simulink model "EPSAC"  (R2016a)
settings: Solver=VariableStepAuto  StartTime=0.0  StopTime=5  RelTol=1e-3
libraries: powerlib x11
settings Model: Creator=jorda  LastModifiedBy=jorda

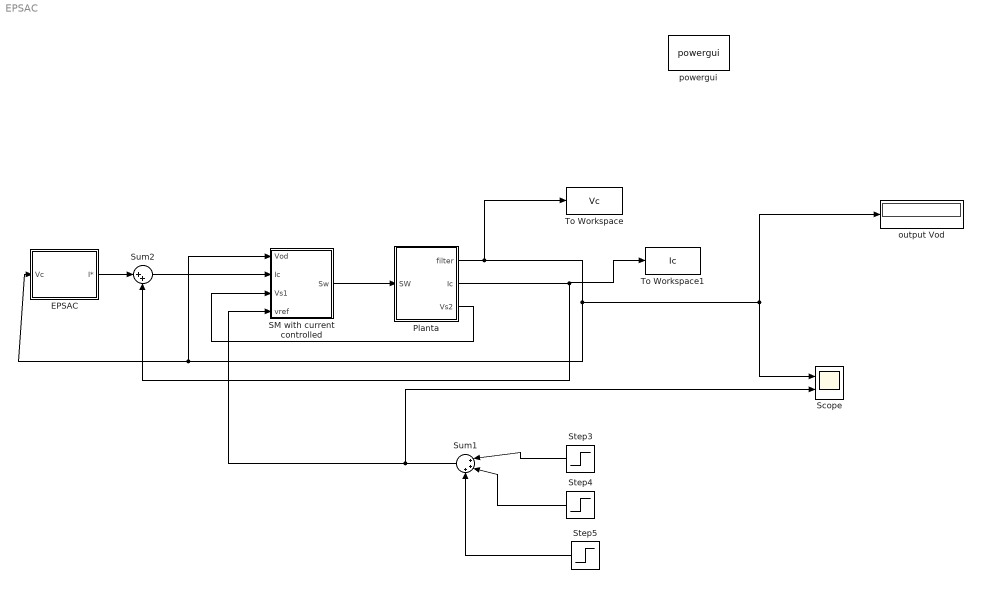
== system EPSAC ==
  EPSAC : Subsystem
  Planta : Subsystem
  SM with current controlled : Subsystem
  Scope : Scope  NumInputPorts=2
  Step3 : Step  Before=20  After=22  SampleTime=0
  Step4 : Step  Time=3  After=-2  SampleTime=0
  Step5 : Step  Time=4  Before=3  After=0  SampleTime=0
  Sum1 : Sum  Inputs=|+++
  Sum2 : Sum  Inputs=|++
  To Workspace : ToWorkspace  VariableName=Vc  SaveFormat=Timeseries  SampleTime=-1
  To Workspace1 : ToWorkspace  VariableName=Ic  SaveFormat=Timeseries  SampleTime=-1
  output Vod : Display
  powergui : powerlib/powergui  Priority=1  SimulationMode=Continuous  SolverType=Tustin/Backward Euler (TBE)  SampleTime=50e-6  frequency=60  SPID=off  DisableSnubberDevices=off  DisableRonSwitches=off  DisableVfSwitches=off  SwTol=0  DisplayEquations=off  Interpol=off  ExternalGateDelay=off  methode=off  Ts=10  FunctionMessages=off  echomessages=off  HookPort=off  EnableUseOfTLC=off  x0status=blocks  frequencyindice=0  Pbase=100e6  ErrMax=1e-4  Iterations=50  UnitsV=kV  UnitsW=MW  buscounter=0  RestoreLinks=warning  ResistiveCurrentMeasurement=off  Frange=[0:2:500]  Ylog=off  Xlog=on  ShowGrid=off  save=off  variable=ZData  structure=0  ZoomFFT=off  StartTime=0.0  cycles=1  DisplayStyle=1  fundamental=60  FreqAxis=off  MaxFrequency=1000  frequencyindicesteady=1  RmsSteady=1  display=off
  wires:
  Step3/1 -> Sum1/1
  Step4/1 -> Sum1/2
  Step5/1 -> Sum1/3
  Planta/3(Vs2) -> SM with current controlled/3("Vs1 ")
  Planta/1(filter) -> To Workspace/1, output Vod/1, Scope/1, EPSAC/1(Vc), SM with current controlled/1(Vod)
  SM with current controlled/1(Sw) -> Planta/1(SW)
  Sum2/1 -> SM with current controlled/2(Ic)
  Sum1/1 -> SM with current controlled/4(vref), Scope/2
  Planta/2(Ic) -> Sum2/2, To Workspace1/1
  EPSAC/1(I*) -> Sum2/1

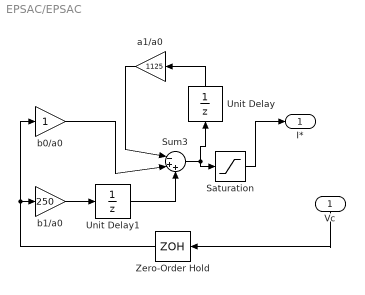
== system EPSAC/EPSAC ==
  Vc : Inport
  Saturation : Saturate  UpperLimit=0.4  LowerLimit=-0.4
  Sum3 : Sum  Inputs=|-++
  Unit Delay : UnitDelay  SampleTime=-1
  Unit Delay1 : UnitDelay  SampleTime=-1
  Zero-Order Hold : ZeroOrderHold  SampleTime=4
  a1/a0 : Gain  Gain=1125
  b0/a0 : Gain
  b1/a0 : Gain  Gain=250
  I* : Outport
  wires:
  Vc/1 -> Zero-Order Hold/1
  Saturation/1 -> I*/1
  b0/a0/1 -> Sum3/2
  Zero-Order Hold/1 -> b0/a0/1, b1/a0/1
  b1/a0/1 -> Unit Delay1/1
  Unit Delay1/1 -> Sum3/3
  a1/a0/1 -> Sum3/1
  Unit Delay/1 -> a1/a0/1
  Sum3/1 -> Saturation/1, Unit Delay/1

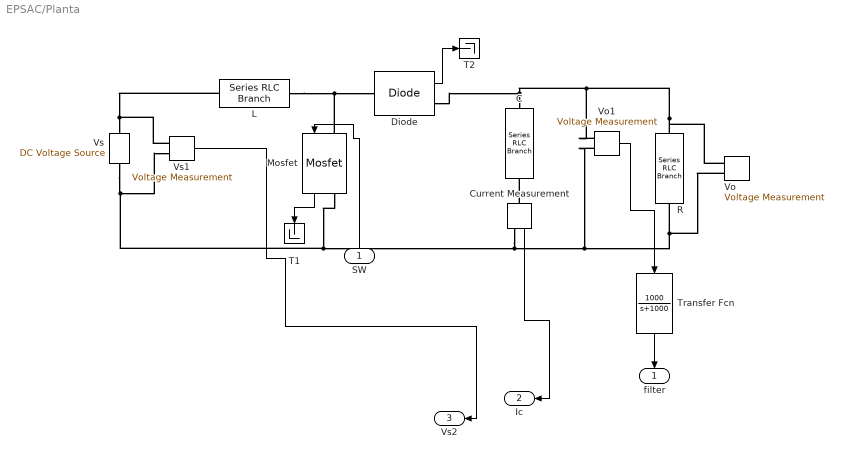
== system EPSAC/Planta ==
  SW : Inport
  C : powerlib/Elements/Series RLC Branch  LConnTagsString=__new0  RConnTagsString=__new0  BranchType=C  Resistance=1  Inductance=1e-3  SetiL0=off  InitialCurrent=0  Capacitance=2000e-6  Setx0=off  InitialVoltage=0  Measurements=None
  Current Measurement : powerlib/Measurements/Current Measurement  PhasorSimulation=off  OutputType=Complex  PSBequivalent=0
  Diode : powerlib/Power Electronics/Diode  Ron=0.001  Lon=0  Vf=0.8  IC=0  UseSnubber=off  Rs=500  Cs=250e-9  Measurements=on
  L : powerlib/Elements/Series RLC Branch  LConnTagsString=__new0  RConnTagsString=__new0  BranchType=L  Resistance=1  Inductance=2e-3  SetiL0=off  InitialCurrent=0  Capacitance=1e-6  Setx0=off  InitialVoltage=0  Measurements=None
  Mosfet : powerlib/Power Electronics/Mosfet  Ron=0.1  Lon=0  Rd=0.01  Vfd=0  IC=0  Rs=1e5  Cs=inf  Measurements=on
  R : powerlib/Elements/Series RLC Branch  LConnTagsString=__new0  RConnTagsString=__new0  BranchType=R  Resistance=4  Inductance=1e-3  SetiL0=off  InitialCurrent=0  Capacitance=1e-6  Setx0=off  InitialVoltage=0  Measurements=None
  T1 : Terminator
  T2 : Terminator
  Transfer Fcn : TransferFcn  Numerator=[1000]  Denominator=[1 1000]
  Vo : powerlib/Measurements/Voltage Measurement  PhasorSimulation=off  OutputType=Complex  PSBequivalent=0
  Vo1 : powerlib/Measurements/Voltage Measurement  PhasorSimulation=off  OutputType=Complex  PSBequivalent=0
  Vs : powerlib/Electrical Sources/DC Voltage Source  Amplitude=15  Measurements=None
  Vs1 : powerlib/Measurements/Voltage Measurement  PhasorSimulation=off  OutputType=Complex  PSBequivalent=0
  filter : Outport
  Ic : Outport  Port=2
  Vs2 : Outport  Port=3
  wires:
  Vo1/1 -> Transfer Fcn/1
  Current Measurement/1 -> Ic/1
  Diode/1 -> T2/1
  Transfer Fcn/1 -> filter/1
  Vs1/1 -> Vs2/1
  Mosfet/1 -> T1/1
  SW/1 -> Mosfet/1
  connections:
  Mosfet/LConn1 -- Diode/LConn1 -- L/RConn1
  L/LConn1 -- Vs1/LConn1 -- Vs/RConn1
  Vs/LConn1 -- Vs1/LConn2 -- Mosfet/RConn1 -- Current Measurement/RConn1 -- Vo1/LConn2 -- R/RConn1 -- Vo/LConn2
  Vo1/LConn1 -- Diode/RConn1 -- C/LConn1 -- R/LConn1 -- Vo/LConn1
  Current Measurement/LConn1 -- C/RConn1

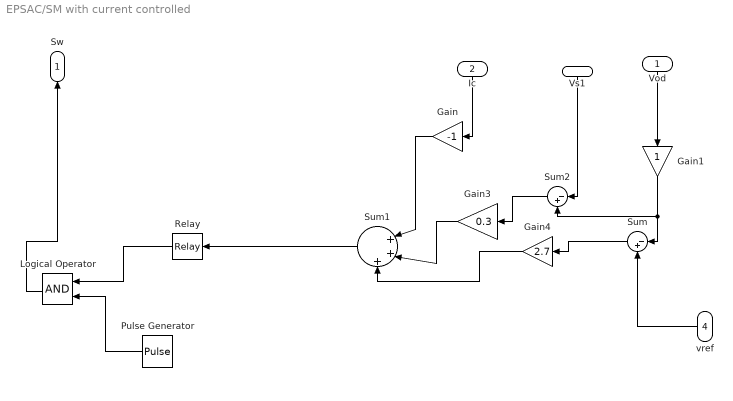
== system EPSAC/SM with current controlled ==
  Vod : Inport
  Ic : Inport  Port=2
  "Vs1 " : Inport  Port=3
  vref : Inport  Port=4
  Gain : Gain  Gain=-1  ParamDataTypeStr=double  OutDataTypeStr=double
  Gain1 : Gain  ParamDataTypeStr=double  OutDataTypeStr=double
  Gain3 : Gain  Gain=0.3  ParamDataTypeStr=double  OutDataTypeStr=double
  Gain4 : Gain  Gain=2.7  ParamDataTypeStr=double  OutDataTypeStr=double
  Logical Operator : Logic  AllPortsSameDT=off  OutDataTypeStr=boolean
  Pulse Generator : DiscretePulseGenerator  PulseType=Time based  Period=1e-3  PulseWidth=50
  Relay : Relay  OnSwitchValue=0.4  OffSwitchValue=-0.4  OutDataTypeStr=Inherit: Inherit via back propagation
  Sum : Sum  Inputs=|-+  AccumDataTypeStr=single  OutDataTypeStr=double  InputSameDT=on
  Sum1 : Sum  Inputs=|+++  AccumDataTypeStr=double  OutDataTypeStr=double  InputSameDT=on
  Sum2 : Sum  Inputs=|-+  AccumDataTypeStr=single  OutDataTypeStr=double  InputSameDT=on
  Sw : Outport
  wires:
  Gain1/1 -> Sum2/2, Sum/1
  "Vs1 "/1 -> Sum2/1
  Vod/1 -> Gain1/1
  Ic/1 -> Gain/1
  vref/1 -> Sum/2
  Sum/1 -> Gain4/1
  Sum2/1 -> Gain3/1
  Gain/1 -> Sum1/1
  Gain3/1 -> Sum1/2
  Gain4/1 -> Sum1/3
  Relay/1 -> Logical Operator/1
  Pulse Generator/1 -> Logical Operator/2
  Logical Operator/1 -> Sw/1
  Sum1/1 -> Relay/1
